simulink model "car_model_PIL"  (R2019b)
settings: Solver=ode23tb  StartTime=0.0  StopTime=30  RelTol=1e-3
InitFcn:
  | CommonVariables
  | Klqr5Velocities
undefined symbols (not defined in the file): A_1, A_2, A_3, A_4, A_5, B1_1, B1_2, B1_3, B1_4, B1_5, BattChrgMax, BattDischrgMax, BrkPrsMax, ChrgLmt_bpt, Disabled, DischrgLmt_bpt, Discovery, disk_abore, DLCXref, DLCYref, efficiency_table, F0z, h, Klqr1, Klqr2, Klqr3, Klqr4, Klqr5, MotSpd, MotTrq, mu_kinetic, Ndiff, num_pads, RegenBrkCutOff, RegenBrkSpd_bpt, Right, Rm, Serial, SOC_bpt, STM32F4, T_eff_bp, VEH, w_eff_bp
libraries: simulink x10, vehdynlibtire x8, vehdynlibsuspension x7, vehdynlibscenariocommon x5, autolibutils x4, sim3dlib x4, autolibmappedmotor x4, autolibshared x2, sharedtransform x2, vehdynlibviscommon x2, pil_lib x1, vehdynlibdriver x1
(part 2 of 7)

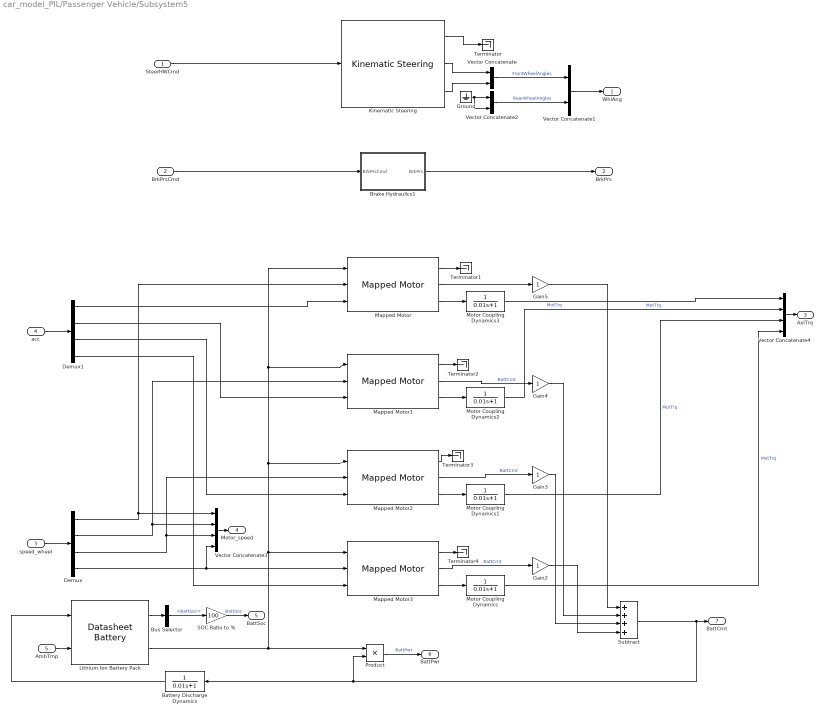
== system car_model_PIL/Passenger Vehicle/Subsystem5 ==
  SteerHWCmd : Inport
  BrkPrsCmd : Inport  Port=2  PortDimensions=4
  speed_wheel : Inport  Port=3
  "acc " : Inport  Port=4
  AmbTmp : Inport  Port=5
  Battery Discharge Dynamics : TransferFcn  Denominator=[0.01 1]
  Brake Hydraulics1 : Subsystem
  Bus Selector : BusSelector  OutputSignals=BattSoc
  Demux : Demux
  Demux1 : Demux
  Gain{2..5} (4 alike) : Gain
  Ground : Ground
  Kinematic Steering : vehdynlibsteering/Kinematic Steering  StrgType=Ackerman  StrgRatioType=Constant  Loc=Front  NrmlFctr=1  TrckWdth=1.922  WhlBase=(1.515+1.504)  Db=0  StrgRng=3*pi  StrgAngBpts="[-6.2832   -5.0265   -3.7699   -2.5133   -1.2566         0    1.2566    2.5133    3.7699    5.0265    6.2832]"  StrgRatioTbl=|  StrgRatio=18  StrgArmLngth=0.1  RckCsLngth=0.5  TieRodLngth=0.248128028933392  D=0.2  PnnRadius=0.0057  PnnRadiusTbl="[0.0055    0.0055    0.0056    0.0057    0.0057    0.0057    0.0057    0.0057    0.0056    0.0055    0.0055]"  RodLngth=0.1  ParaArmLngth=0.9  aMode=2
      | [13.5000   13.3750   13.2500   13.1250   13.0000   13.0000   13.0000   13.1250   13.2500   13.3750   13.5000
      | ]
      settings: SourceProductName=Vehicle Dynamics Blockset
  Lithium Ion Battery Pack : autolibdatasheetbattery/Datasheet Battery  CapacityCtrl=Parameter  OutputVlt=Unfiltered  BattChargeMax=BattChargeMax  Em=Em  CapLUTBp=CapLUTBp  RInt=RInt  BattTempBp=BattTempBp  CapSOCBp=CapSOCBp  Ns=Ns  Np=Np  BattCapInit=BattCapInit  Tc=1/1000  Vinit=3.75*72  RefBlkName='autolibdatasheetbattery/Datasheet Battery'
      settings: SourceProductName=Powertrain Blockset  SourceProductBaseCode=PW
  Mapped Motor{,1..3} (4 alike) : autolibmappedmotor/Mapped Motor  port_config=Speed  param_by=Maximum torque and power  w_t=[ 0 375 750 800 ]  T_t=[0.09 0.08 0.07 0]  torque_max=torque_max  power_max=power_max  Tc=Tc  param_loss=Tabulated efficiency data  eff=100  w_eff=375  T_eff=0.08  Piron=0  Pbase=0  w_eff_bp=w_eff_bp.*pi/30  T_eff_bp=T_eff_bp  Temp_eff_bp=[233.15 293.15 373.15]  losses_table=[1 2;3 4]  losses_table_3d=cat(3,[1.49 1.67 2.21 3.10; 0.42 0.69 1.14 2.03; 0.06 0.24 0.78 1.68; 0.42 0.69 1.14 2.03; 1.49 1.67 2.21 3.10],[1.49 1.67 2.21 3.10; 0.42 0.69 1.14 2.03; 0.06 0.24 0.78 1.68; 0.42 0.69 1.14 2.03; 1.49 1.67 2.21 3.10],[1.49 1.67 2.21 3.10; 0.42 0.69 1.14 2.03; 0.06 0.24 0.78 1.68; 0.42 0.69 1.14 2.03; 1.49 1.67 2.21 3.10])  efficiency_table=efficiency_table  efficiency_table_3d=cat(3,[95 95 95 95; 95 95 95 95; 95 95 95 95; 95 95 95 95; 95 95 95 95],[95 95 95 95; 95 95 95 95; 95 95 95 95; 95 95 95 95; 95 95 95 95],[95 95 95 95; 95 95 95 95; 95 95 95 95; 95 95 95 95; 95 95 95 95])  J=5e-6  b=1e-5  omega_o=0  T_t_extended=[0 0.07 0.08 0.09 0.08 0.07 0]  w_t_extended=[-800 -750 -375 0 375 750 800]  KLossIron=0  KLossCopper=0  x_w_eff_vec=[-1047.1975511966 -942.477796076938 -837.758040957278 -733.038285837618 -628.318530717959 -523.598775598299 -418.879020478639 -314.159265358979 -285.714285713875 -209.43951023932 -104.71975511966 0 104.71975511966 209.43951023932 285.714285713875 314.159265358979 418.879020478639 523.598775598299 628.318530717959 733.038285837618 837.758040957278 942.477796076938 1047.1975511966]  x_T_eff_vec=[-280 -260 -240 -220 -200 -180 -160 -140 -120 -100 -80 -60 -40 -20 0 20 40 60 80 100 120 140 160 180 200 220 240 260 280]  x_tmp_eff_vec=[-0.09 -0.06 -0.03 0 0.03 0.06 0.09]  x_losses_mat=[22069.9698961863 20493.5434750302 18917.117053874 17340.6906327178 15764.2642115617 14187.8377904055 12611.4113692493 11034.9849480932 9458.558526937 7882.13210578084 6305.70568462467 5463.63939754746 4654.21133865155 3695.99135716446 0 3141.59265358979 4188.79020478639 5026.54824574367 5864.30628670094 7330.38285837618 8796.45943005141 10262.5360017267 11728.6125734019 13194.6891450771 14660.7657167524 16126.8422884276 17592.9188601028 19058.9954317781 20525.0720034533;16844.2840149921 15641.1208710641 14437.9577271361 13234.7945832081 12031.6314392801 10828.4682953521 9625.30515142405 8422.14200749604 7218.97886356803 6015.81571964003 4812.65257571202 3609.48943178402 2837.5675580811 3326.39222144802 0 2827.43338823081 2638.93782901542 3392.92006587697 4523.8934211693 5654.86677646162 6785.84013175395 7916.81348704627 9047.7868423386 10178.7601976309 11309.7335529232 12440.7069082156 13571.6802635079 14702.6536188002 15833.6269740925;12345.907972002 11464.0574025733 10582.2068331446 9700.35626371584 8818.50569428713 7936.65512485842 7054.8045554297 6172.95398600099 5291.10341657228 4409.25284714356 3527.40227771485 3208.43505047468 2522.28227384987 2956.79308573157 0 2513.27412287184 2345.72251468038 3015.9289474462 3351.03216382911 4188.79020478639 5026.54824574366 5864.30628670094 6702.06432765822 7539.82236861549 8377.58040957277 9215.33845053005 10053.0964914873 10890.8545324446 11728.6125734019;10802.6694755017 10031.0502272516 9259.43097900148 8487.81173075136 7716.19248250124 6944.57323425111 6172.95398600099 5401.33473775087 4629.71548950074 3858.09624125062 3086.47699300049 2807.38066916535 2206.99698961863 2587.19395001512 0 2199.11485751286 2052.50720034533 2638.93782901542 2932.15314335047 3665.19142918809 4398.2297150257 5131.26800086332 5864.30628670094 6597.34457253856 7330.38285837617 8063.42114421379 8796.45943005141 9529.49771588903 10262.5360017266;9259.43097900149 8598.04305192995 7936.65512485842 7275.26719778688 6613.87927071535 5952.49134364381 5291.10341657228 4629.71548950074 3968.32756242921 3306.93963535767 3208.43505047468 2406.32628785601 1891.7117053874 2217.59481429868 0 1884.95559215388 1759.29188601028 2261.94671058465 3015.9289474462 3141.59265358979 3769.91118430775 4398.22971502571 5026.54824574366 5654.86677646162 6283.18530717958 6911.50383789754 7539.82236861549 8168.14089933345 8796.45943005141;7716.19248250124 7165.03587660829 6613.87927071535 6062.7226648224 5511.56605892946 4960.40945303651 4409.25284714356 3858.09624125062 3306.93963535767 2755.78302946473 2673.69587539557 2005.27190654668 1576.42642115617 1847.99567858223 0 1570.7963267949 1466.07657167524 1884.95559215387 2513.27412287183 2617.99387799149 3141.59265358979 3665.19142918809 4188.79020478639 4712.38898038468 5235.98775598298 5759.58653158128 6283.18530717958 6806.78408277788 7330.38285837618;7486.34845110759 6951.60927602848 6416.87010094936 5882.13092587025 5347.39175079114 4812.65257571202 4277.91340063291 3743.17422555379 3208.43505047468 2673.69587539557 2138.95670031645 1604.21752523734 1261.14113692493 1478.39654286579 0 1256.63706143592 1172.86125734019 1507.9644737231 2010.61929829747 2513.27412287183 3015.9289474462 3518.58377202056 4021.23859659493 4523.8934211693 5026.54824574366 5529.20307031803 6031.8578948924 6534.51271946676 7037.16754404113;9773.84381116825 9075.71211037052 8377.58040957279 7679.44870877505 5463.63939754746 4917.27545779272 4370.91151803797 3310.49548442795 2837.5675580811 2364.63963173425 1891.7117053874 1639.09181926424 1092.72787950949 1108.79740714934 0 942.477796076938 1005.30964914873 1507.9644737231 1759.29188601028 2199.11485751285 2638.93782901542 3078.760800518 4021.23859659493 4523.8934211693 5026.54824574367 6911.50383789754 7539.8223686155 8168.14089933346 8796.45943005142;8888.88888887612 8253.9682539564 7619.04761903668 6984.12698411695 4968.94409937174 4472.04968943457 3975.15527949739 3478.26086956022 2981.36645962304 2484.47204968587 1987.5776397487 ...(+6498 chars)]  x_losses_mat_3d=[37.8947368421052 25.2631578947368 12.6315789473684 0 12 24 36;18.9473684210526 12.6315789473684 6.3157894736842 0 5.99999999999999 12 18;0 0 0 0 0 0 0;18 12 5.99999999999999 0 6.3157894736842 12.6315789473684 18.9473684210526;36 24 12 0 12.6315789473684 25.2631578947368 37.8947368421052]  CalLossMapData={}  CalLossWithTempMapData={}  aMode=aMode  RefBlkName='autolibmappedmotor/Mapped Motor'
      settings: SourceProductName=Powertrain Blockset  SourceProductBaseCode=PW
  Motor Coupling Dynamics{,1..3} (4 alike) : TransferFcn  Denominator=[0.01 1]
  Product : Product
  SOC Ratio to % : Gain  Gain=100
  Subtract : Sum  Inputs=++++
  Terminator{,1..4} (5 alike) : Terminator
  Vector Concatenate : Concatenate
  Vector Concatenate1 : Concatenate
  Vector Concatenate2 : Concatenate
  Vector Concatenate3 : Concatenate  NumInputs=4
  Vector Concatenate4 : Concatenate  NumInputs=4
  WhlAng : Outport  Unit=rad  VectorParamsAs1DForOutWhenUnconnected=off
  BrkPrs : Outport  Port=2  PortDimensions=4  VectorParamsAs1DForOutWhenUnconnected=off
  AxlTrq : Outport  Port=3  VectorParamsAs1DForOutWhenUnconnected=off
  Motor_speed : Outport  Port=4  VectorParamsAs1DForOutWhenUnconnected=off
  BattSoc : Outport  Port=5  VectorParamsAs1DForOutWhenUnconnected=off
  BattPwr : Outport  Port=6  VectorParamsAs1DForOutWhenUnconnected=off
  BattCrnt : Outport  Port=7  VectorParamsAs1DForOutWhenUnconnected=off
  wires:
  SteerHWCmd/1 -> Kinematic Steering/1
  Kinematic Steering/1 -> Terminator/1
  Vector Concatenate2/1 -> Vector Concatenate1/2  "RearWheelAngles"
  Vector Concatenate1/1 -> WhlAng/1
  BrkPrsCmd/1 -> Brake Hydraulics1/1(BrkPrsCmd)
  Brake Hydraulics1/1(BrkPrs) -> BrkPrs/1
  Kinematic Steering/2 -> Vector Concatenate/1
  Kinematic Steering/3 -> Vector Concatenate/2
  Vector Concatenate/1 -> Vector Concatenate1/1  "FrontWheelAngles"
  Mapped Motor3/3 -> Motor Coupling Dynamics/1
  Battery Discharge Dynamics/1 -> Lithium Ion Battery Pack/1
  Product/1 -> BattPwr/1  "BattPwr"
  Motor Coupling Dynamics/1 -> Vector Concatenate4/4  "MotTrq"
  AmbTmp/1 -> Lithium Ion Battery Pack/2
  SOC Ratio to %/1 -> BattSoc/1  "BattSoc"
  Lithium Ion Battery Pack/2 -> Product/1, Mapped Motor3/1, Mapped Motor2/1, Mapped Motor1/1, Mapped Motor/1
  Demux1/4 -> Mapped Motor3/3
  Demux1/3 -> Mapped Motor2/3
  Mapped Motor2/3 -> Motor Coupling Dynamics1/1
  Motor Coupling Dynamics1/1 -> Vector Concatenate4/3  "MotTrq"
  Demux1/2 -> Mapped Motor1/3
  Motor Coupling Dynamics2/1 -> Vector Concatenate4/2  "MotTrq"
  Demux1/1 -> Mapped Motor/3
  Motor Coupling Dynamics3/1 -> Vector Concatenate4/1  "MotTrq"
  Vector Concatenate4/1 -> AxlTrq/1
  Subtract/1 -> Product/2, Battery Discharge Dynamics/1, BattCrnt/1
  Mapped Motor2/2 -> Gain3/1  "BattCrnt"
  Mapped Motor1/2 -> Gain4/1  "BattCrnt"
  Mapped Motor3/2 -> Gain2/1  "BattCrnt"
  Gain2/1 -> Subtract/4
  Gain3/1 -> Subtract/3
  Gain4/1 -> Subtract/2
  Gain5/1 -> Subtract/1
  "acc "/1 -> Demux1/1
  Mapped Motor/1 -> Terminator1/1
  Mapped Motor/3 -> Motor Coupling Dynamics3/1
  Mapped Motor/2 -> Gain5/1
  Mapped Motor1/3 -> Motor Coupling Dynamics2/1
  Mapped Motor1/1 -> Terminator2/1
  Mapped Motor2/1 -> Terminator3/1
  Mapped Motor3/1 -> Terminator4/1
  Vector Concatenate3/1 -> Motor_speed/1
  speed_wheel/1 -> Demux/1
  Demux/1 -> Mapped Motor/2, Vector Concatenate3/1
  Demux/2 -> Vector Concatenate3/2, Mapped Motor1/2
  Demux/3 -> Mapped Motor2/2, Vector Concatenate3/3
  Demux/4 -> Vector Concatenate3/4, Mapped Motor3/2
  Lithium Ion Battery Pack/1 -> Bus Selector/1
  Bus Selector/1 -> SOC Ratio to %/1  "<BattSoc>"
  Ground/1 -> Vector Concatenate2/2, Vector Concatenate2/1

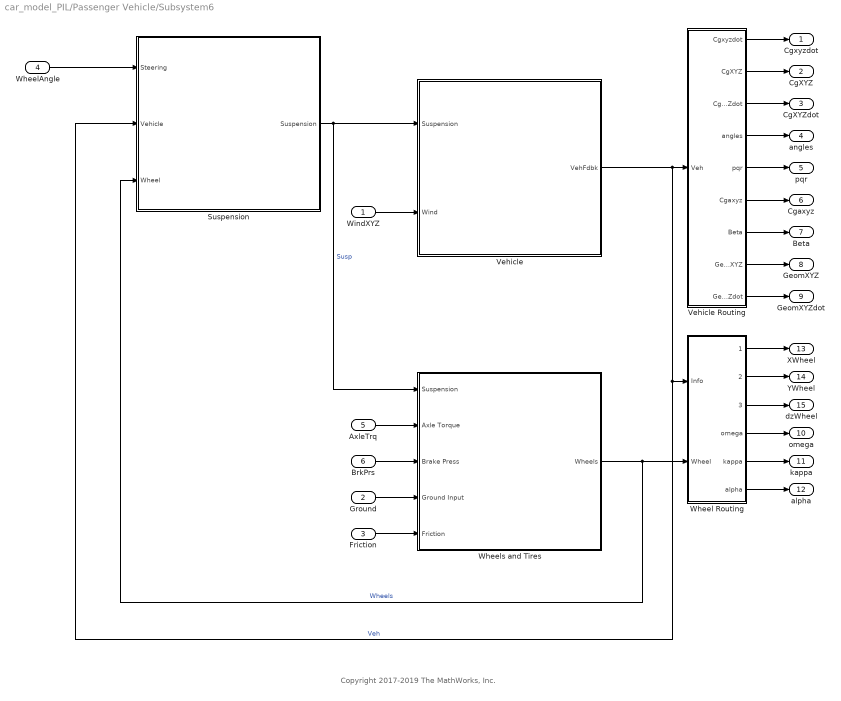
== system car_model_PIL/Passenger Vehicle/Subsystem6 ==
  note: Copyright 2017-2019 The MathWorks, Inc.
  WindXYZ : Inport  Unit=m/s  PortDimensions=3
  Ground : Inport  Port=2  Unit=m  PortDimensions=4
  Friction : Inport  Port=3  Unit=1  PortDimensions=4
  WheelAngle : Inport  Port=4  Unit=rad  PortDimensions=4
  AxleTrq : Inport  Port=5  Unit=N*m  PortDimensions=4
  BrkPrs : Inport  Port=6  PortDimensions=4
  Suspension : Subsystem  VariantControlMode=Label  Variant=on  LabelModeActiveChoice=3
      mask Display:
      | switch str2num(get_param(gcb,'ActiveVariant'))
      |     case 1
      |         image('suspdw.png');
      |     case 2
      |         image([imread('suspindmap.png');imread('suspsamap.png')]);
      |     case 3
      |          image([imread('suspmacp.png');imread('suspsacoil.png')]);
      |     case 4
      |          image('suspmacp.png');
      |     case 5
      |          image('suspindmap.png');
      | end
  Vehicle : Subsystem
      mask Display: image('6dofcar.png');
  Vehicle Routing : Subsystem
  Wheel Routing : Subsystem
  Wheels and Tires : Subsystem
      mask Display: image('wheel3dof.png')
  Cgxyzdot : Outport  VectorParamsAs1DForOutWhenUnconnected=off
  CgXYZ : Outport  Port=2  VectorParamsAs1DForOutWhenUnconnected=off
  CgXYZdot : Outport  Port=3  VectorParamsAs1DForOutWhenUnconnected=off
  angles : Outport  Port=4  VectorParamsAs1DForOutWhenUnconnected=off
  pqr : Outport  Port=5  VectorParamsAs1DForOutWhenUnconnected=off
  Cgaxyz : Outport  Port=6  VectorParamsAs1DForOutWhenUnconnected=off
  Beta : Outport  Port=7  VectorParamsAs1DForOutWhenUnconnected=off
  GeomXYZ : Outport  Port=8  VectorParamsAs1DForOutWhenUnconnected=off
  GeomXYZdot : Outport  Port=9  VectorParamsAs1DForOutWhenUnconnected=off
  omega : Outport  Port=10  PortDimensions=4  VectorParamsAs1DForOutWhenUnconnected=off
  kappa : Outport  Port=11  PortDimensions=4  VectorParamsAs1DForOutWhenUnconnected=off
  alpha : Outport  Port=12  PortDimensions=4  VectorParamsAs1DForOutWhenUnconnected=off
  XWheel : Outport  Port=13  VectorParamsAs1DForOutWhenUnconnected=off
  YWheel : Outport  Port=14  VectorParamsAs1DForOutWhenUnconnected=off
  dzWheel : Outport  Port=15  PortDimensions=4  VectorParamsAs1DForOutWhenUnconnected=off
  wires:
  Vehicle Routing/7(Beta) -> Beta/1
  Vehicle/1(VehFdbk) -> Suspension/2(Vehicle), Wheel Routing/1(Info), Vehicle Routing/1(Veh)  "Veh"
  Friction/1 -> Wheels and Tires/5(Friction)
  WheelAngle/1 -> Suspension/1(Steering)
  WindXYZ/1 -> Vehicle/2(Wind)
  Wheels and Tires/1(Wheels) -> Suspension/3(Wheel), Wheel Routing/2(Wheel)  "Wheels"
  Vehicle Routing/2(CgXYZ) -> CgXYZ/1
  AxleTrq/1 -> Wheels and Tires/2(Axle Torque)
  Vehicle Routing/4(angles) -> angles/1
  Wheel Routing/1(XWheel) -> XWheel/1
  Vehicle Routing/1(Cgxyzdot) -> Cgxyzdot/1
  Wheel Routing/2(YWheel) -> YWheel/1
  Suspension/1(Suspension) -> Wheels and Tires/1(Suspension), Vehicle/1(Suspension)  "Susp"
  Wheel Routing/4(omega) -> omega/1
  Vehicle Routing/6(Cgaxyz) -> Cgaxyz/1
  Vehicle Routing/5(pqr) -> pqr/1
  BrkPrs/1 -> Wheels and Tires/3(Brake Press)
  Vehicle Routing/8(GeomXYZ) -> GeomXYZ/1
  Vehicle Routing/9(GeomXYZdot) -> GeomXYZdot/1
  Ground/1 -> Wheels and Tires/4(Ground Input)
  Wheel Routing/3(ZWheel) -> dzWheel/1
  Wheel Routing/5(kappa) -> kappa/1
  Vehicle Routing/3(CgXYZdot) -> CgXYZdot/1
  Wheel Routing/6(alpha) -> alpha/1

== system car_model_PIL/Reference Generator/3D Engine ==
  note: 1) Add Subsystem or Model blocks as valid variant choices.
      | 2) You cannot connect blocks at this level. At simulation, connectivity is automatically
      | determined, based on the active variant and port name matching.
  VehFdbk : Inport
  3D Engine : Subsystem  VariantControl=1
  3D Engine Disabled : Subsystem  VariantControl=0

== system car_model_PIL/Reference Generator/Reference Generator ==
  "VehFdbk " : Inport
  Constant Radius : Subsystem  AncestorBlock=vehdynlibscenariocommon/Constant Radius  VariantControl=4  mask{t_start=t_start, xdot_r=xdot_r, xdotUnit=mph, R=R, turnDirMask=Right, ay_max=cr_ay_max, ay_stop=off, Parameter6=2}
      mask prompts: t_start "Maneuver start time, t_start [s]:"; xdot_r "Longitudinal velocity reference, xdot_r:"; xdotUnit "Longitudinal velocity reference units, xdotUnit []:"; R "Radius value, R [m]:"; turnDirMask "Turn direction"; ay_max "Lateral acceleration absolute threshold, ay_max [g]:"; ay_stop "Stop simulation at lateral acceleration threshold"
      mask TypeOptions xdotUnit: Longitudinal Velocity Reference/Input Units/Unit
      mask TypeOptions R: Constant Radius/Value
      mask TypeOptions turnDirMask: Constant Radius/turnDirMask
  Double Lane Change : Subsystem  VariantControl=0
  Increasing Steer : Subsystem  VariantControl=1
  Sine with Dwell : Subsystem  VariantControl=3
  Swept Sine : Subsystem  VariantControl=2
  " Vis" : Outport  VectorParamsAs1DForOutWhenUnconnected=off
  " Ref" : Outport  Port=2  VectorParamsAs1DForOutWhenUnconnected=off
  " Fdbk" : Outport  Port=3  VectorParamsAs1DForOutWhenUnconnected=off

== system car_model_PIL/Visualization/ISO 15037-1:2006 ==
  VehFdbk : Inport
  Cntrl : Inport  Port=2
  Disabled : Subsystem  VariantControl=0
  Enabled : Subsystem  VariantControl=1

== system car_model_PIL/Visualization/Scope Type ==
  "VehFdbk " : Inport
  Cntrl : Inport  Port=2
  "Vis " : Inport  Port=3
  DLC : Subsystem  VariantControl=1
  None : Subsystem  VariantControl=0
  XYZ : Subsystem  VariantControl=2
  " Ref" : Outport  VectorParamsAs1DForOutWhenUnconnected=off

== system car_model_PIL/Visualization/Vehicle XY Plotter ==
  "VehFdbk " : Inport
  "Ref " : Inport  Port=2
  XY View : Subsystem  VariantControl=0
  XY View Ref : Subsystem  VariantControl=1

== system car_model_PIL/Controllers/Accel Pedal to Traction Wheel Torque Request/Apply ESP control ==
  Beta : Inport
  Omega : Inport  Port=2
  Vspd : Inport  Port=3
  K1 : Gain  Gain=Klqr1  Multiplication=Matrix(K*u)
  K2 : Gain  Gain=Klqr2  Multiplication=Matrix(K*u)
  K3 : Gain  Gain=Klqr3  Multiplication=Matrix(K*u)
  K4 : Gain  Gain=Klqr4  Multiplication=Matrix(K*u)
  K5 : Gain  Gain=Klqr5  Multiplication=Matrix(K*u)
  Switch control action : MATLAB Function  TreatAsAtomicUnit=on
  Vector Concatenate : Concatenate
  dWhlSpd : Outport
  wires:
  Beta/1 -> Vector Concatenate/1
  Vector Concatenate/1 -> Switch control action/7(x), K5/1, K4/1, K3/1, K2/1, K1/1
  K5/1 -> Switch control action/6(contr5)
  Omega/1 -> Vector Concatenate/2
  K1/1 -> Switch control action/2(contr1)
  K3/1 -> Switch control action/4(contr3)
  K4/1 -> Switch control action/5(contr4)
  K2/1 -> Switch control action/3(contr2)
  Vspd/1 -> Switch control action/1(V)
  Switch control action/1(u) -> dWhlSpd/1

== system car_model_PIL/Controllers/Accel Pedal to Traction Wheel Torque Request/Signals to states ==
  Beta : Inport
  YawRate : Inport  Port=2
  WhlAng : Inport  Port=3
  Vspd : Inport  Port=4
  Constant : Constant  Value=[A_1;A_2;A_3;A_4;A_5]  VectorParams1D=off
  Constant1 : Constant  Value=[B1_1;B1_2;B1_3;B1_4;B1_5]  VectorParams1D=off
  Demux : Demux  Outputs=2
  Gain : Gain  Gain=1/2
  Subtract : Sum  Inputs=+-
  Subtract1 : Sum  Inputs=-+
  Sum of Elements : Sum  Inputs=+
  equilibrium point : MATLAB Function  TreatAsAtomicUnit=on
  Beta_state : Outport
  Omega_state : Outport  Port=2
  wires:
  Subtract/1 -> Beta_state/1
  Beta/1 -> Subtract/1
  Subtract1/1 -> Omega_state/1
  YawRate/1 -> Subtract1/2
  WhlAng/1 -> Sum of Elements/1
  Sum of Elements/1 -> Gain/1
  equilibrium point/1(x_eq) -> Demux/1
  Demux/1 -> Subtract/2
  Demux/2 -> Subtract1/1
  Gain/1 -> equilibrium point/1(delta)
  Vspd/1 -> equilibrium point/2(V)
  Constant/1 -> equilibrium point/3(A_mat)
  Constant1/1 -> equilibrium point/4(B_mat)

== system car_model_PIL/Controllers/Accel Pedal to Traction Wheel Torque Request/Virtual Ackerman differential ==
  note: Wheels are organized as:
      |
      | 1 ------------ 2
      | |
      | |
      | |
      | |
      | 3 ------------ 4
      |
      | But output inverting 3 and 4
      | (for easier integration)
  WhlAng : Inport
  RefSpd : Inport  Port=2
  Abs : Abs
  Cos : Trigonometry  Operator=cos
  Demux : Demux
  Divide : Product  Inputs=*/
  Divide1 : Product  Inputs=*/
  Divide2 : Product  Inputs=*/
  Fcn : Fcn  Expr=sqrt( ((u(4) + u(5))/ 2)^2 + u(1)^2 )
  Mux : Mux
  Product : Product
  Product1 : Product
  Saturation RefSpd : Saturate  UpperLimit=120  LowerLimit=-120
  Saturation WhlAnd : Saturate  UpperLimit=pi*5/12  LowerLimit=-pi*5/12
  Saturation WhlSpd : Saturate  UpperLimit=600  LowerLimit=-600
  Sin : Trigonometry
  Sum : Sum  Inputs=+-|
  Vector Concatenate1 : Concatenate
  Vector Concatenate2 : Concatenate
  pi half : Constant  Value=pi/2
  wheel base : Constant  Value=VEH.FrontAxlePositionfromCG+VEH.RearAxlePositionfromCG
  wheel base1 : Constant  Value=VEH.RearAxlePositionfromCG
  wheel radius : Constant  Value=VEH.WheelRadius
  WhlSpd : Outport
  wires:
  Sin/1 -> Product1/2
  Cos/1 -> Divide/2
  wheel base/1 -> Divide/1
  Divide/1 -> Vector Concatenate2/1, Product1/1  "[d1; d2]"
  Vector Concatenate1/1 -> Fcn/1
  Fcn/1 -> Divide1/2  "d_v"
  Divide1/1 -> Product/1  "w_v"
  Divide2/1 -> Product/2  "d_x/r_w"
  wheel radius/1 -> Divide2/2
  pi half/1 -> Sum/1
  Sum/1 -> Sin/1, Cos/1
  Product1/1 -> Vector Concatenate2/2  "[d3; d4]"
  Vector Concatenate2/1 -> Divide2/1, Vector Concatenate1/2  "[d1; d2; d3; d4]"
  Abs/1 -> Sum/2
  Saturation WhlAnd/1 -> Abs/1
  WhlAng/1 -> Saturation WhlAnd/1  "[delta1; delta2]"
  Saturation RefSpd/1 -> Divide1/1
  RefSpd/1 -> Saturation RefSpd/1
  Product/1 -> Saturation WhlSpd/1  "[w1; w2; w3; w4]"
  Saturation WhlSpd/1 -> Demux/1
  Mux/1 -> WhlSpd/1
  Demux/1 -> Mux/1
  Demux/2 -> Mux/2
  Demux/4 -> Mux/3
  Demux/3 -> Mux/4
  wheel base1/1 -> Vector Concatenate1/1

== system car_model_PIL/Controllers/Accel Pedal to Traction Wheel Torque Request1/__InputSSForSFun__ ==
  AccelPdl : Inport
  WhlAng : Inport  Port=2
  xdot : Inport  Port=3
  ydot : Inport  Port=4
  YawRate : Inport  Port=5
  MotSpd : Inport  Port=6
  __UniqueOutportName__1__ : Outport
  __UniqueOutportName__2__ : Outport  Port=2
  __UniqueOutportName__3__ : Outport  Port=3
  __UniqueOutportName__4__ : Outport  Port=4
  __UniqueOutportName__5__ : Outport  Port=5
  __UniqueOutportName__6__ : Outport  Port=6
  wires:
  AccelPdl/1 -> __UniqueOutportName__1__/1
  WhlAng/1 -> __UniqueOutportName__2__/1
  xdot/1 -> __UniqueOutportName__3__/1
  ydot/1 -> __UniqueOutportName__4__/1
  YawRate/1 -> __UniqueOutportName__5__/1
  MotSpd/1 -> __UniqueOutportName__6__/1

== system car_model_PIL/Controllers/Accel Pedal to Traction Wheel Torque Request1/__OutputSSForSFun__ ==
  __UniqueInportName__1__ : Inport
  TrqCmd : Outport  VectorParamsAs1DForOutWhenUnconnected=off
  wires:
  __UniqueInportName__1__/1 -> TrqCmd/1

== system car_model_PIL/Controllers/Motor Torque Arbitration and Power Management/Power Management ==
  note: Power Management algorithm:
      | - Estimate Elec power based on mech power using efficiency map
      | - Check if Elec power is within battery power limits
      | - If power within limit , use motor torque command
      | - If power limit exceeded, use limited motor torque
      | - For low Mot Spd, MotPwrReq will be a small number.  Pass through torque command until Mot Spd > 2.
  BattPwrDischrgLmt : Inport
  BattPwrChrgLmt : Inport  Port=2
  MotSpd : Inport  Port=3
  MotTrqCmd : Inport  Port=4
  Abs : Abs
  Check Within Limits : Subsystem
  Compare To Constant : simulink/Logic and Bit Operations/Compare To Constant  relop=<  const=2  OutDataTypeStr=boolean
  ElecToMechPwr : Product  Inputs=*/
  Mech to Elec Power Estimate : Subsystem
  MechPwrToTrq : Product  Inputs=*/
  Switch : Switch  Criteria=u2 > Threshold
  Switch1 : Switch  Criteria=u2 > Threshold
  Torque Limit : Subsystem
  div0protect - poly : autolibutils/div0protect - poly  thresh=2  aMode=aMode
      settings: SourceProductName=Powertrain Blockset  SourceProductBaseCode=PW
  MotTrqCmdFinal : Outport  VectorParamsAs1DForOutWhenUnconnected=off
  wires:
  MotSpd/1 -> Abs/1, Torque Limit/2(MotSpd), div0protect - poly/1, Mech to Elec Power Estimate/2(MotSpd)
  MotTrqCmd/1 -> Switch/1, Switch1/1, Mech to Elec Power Estimate/1(MotTrqCmd)
  div0protect - poly/1 -> MechPwrToTrq/2
  Mech to Elec Power Estimate/2(Eff2k) -> ElecToMechPwr/2
  ElecToMechPwr/1 -> MechPwrToTrq/1
  MechPwrToTrq/1 -> Switch/3
  Torque Limit/1(MotTrqCmd) -> MotTrqCmdFinal/1
  BattPwrDischrgLmt/1 -> Check Within Limits/1(up)
  Mech to Elec Power Estimate/1(MotPwrElecReq) -> Check Within Limits/2(u)
  BattPwrChrgLmt/1 -> Check Within Limits/3(lo)
  Check Within Limits/2(y) -> ElecToMechPwr/1
  Switch/1 -> Switch1/3
  Check Within Limits/1(InLimit) -> Switch/2
  Switch1/1 -> Torque Limit/1(MotTrq)
  Abs/1 -> Compare To Constant/1
  Compare To Constant/1 -> Switch1/2

== system car_model_PIL/Controllers/Regen Braking Control/Parallel Regen Braking ==
  VehSpd : Inport
  MotSpd : Inport  Port=2
  "BrkPrsReq " : Inport  Port=3
  BattSoc : Inport  Port=4
  ChrgLmt : Lookup_n-D  NumberOfTableDimensions=1  BreakpointsForDimension1=[0:10:100]  Table=[1 1 1 1 1 1 1 1 0.7 0.35 0]  ExtrapMethod=Clip  UseLastTableValue=on  InternalRulePriority=Speed  RndMeth=Simplest  InputSameDT=on
  Gain : Gain  Gain=-1
  MaxMotorTrqVsSpd : Lookup_n-D  NumberOfTableDimensions=1  BreakpointsForDimension1=MotSpd  Table=MotTrq  ExtrapMethod=Clip  UseLastTableValue=on  InternalRulePriority=Speed  OutDataTypeStr=Inherit: Inherit from 'Table data'  RndMeth=Simplest  InputSameDT=on
  Product1 : Product
  Product3 : Product
  RegenBrakingCutoff : Lookup_n-D  NumberOfTableDimensions=1  BreakpointsForDimension1=[2.2 4.5]  Table=[0 1]  ExtrapMethod=Clip  UseLastTableValue=on  InternalRulePriority=Speed  RndMeth=Simplest  InputSameDT=on
  rads_to_rpm : Gain  Gain=30/pi
  " MotTrqCmdRegen" : Outport  VectorParamsAs1DForOutWhenUnconnected=off
  " BrkCmd" : Outport  Port=2  VectorParamsAs1DForOutWhenUnconnected=off
  wires:
  Gain/1 -> " MotTrqCmdRegen"/1
  BattSoc/1 -> ChrgLmt/1
  Product3/1 -> Gain/1  "MotTrqRegen"
  Product1/1 -> Product3/2  "RegenFactor"
  RegenBrakingCutoff/1 -> Product1/1
  VehSpd/1 -> RegenBrakingCutoff/1
  ChrgLmt/1 -> Product1/2
  MaxMotorTrqVsSpd/1 -> Product3/1  "MotTrqMax"
  rads_to_rpm/1 -> MaxMotorTrqVsSpd/1
  MotSpd/1 -> rads_to_rpm/1
  "BrkPrsReq "/1 -> " BrkCmd"/1  "BrkPrsReq"

== system car_model_PIL/Controllers/Regen Braking Control/Series Regen Braking ==
  note: - Total brake torque request based on brake pressure and parameters of disc brakes
      | - Use as much regenerative motor braking as possible
      | - Any braking torque request that cannot be provided by the motor, will be provided by the friction brakes
  note: T / 4 brakes*(muk*pi*Ba^2*Rm*Npads/4)
  note: 4 brakes*(muk*pi*Ba^2*Rm*Npads/4)*P
  VehSpd : Inport
  MotSpd : Inport  Port=2
  "BrkPrsReq " : Inport  Port=3
  BattSoc : Inport  Port=4
  ChrgLmt : Lookup_n-D  NumberOfTableDimensions=1  BreakpointsForDimension1=SOC_bpt  Table=ChrgLmt_bpt  ExtrapMethod=Clip  UseLastTableValue=on  InternalRulePriority=Speed  RndMeth=Simplest  InputSameDT=on
  Constant : Constant  Value=4*(mu_kinetic*pi*disk_abore^2*Rm*num_pads/4)
  Constant1 : Constant  Value=4*(mu_kinetic*pi*disk_abore^2*Rm*num_pads/4)
  Gain : Gain  Gain=-1
  MaxMotTrqVsSpd : Lookup_n-D  NumberOfTableDimensions=1  BreakpointsForDimension1=MotSpd  Table=MotTrq  ExtrapMethod=Clip  UseLastTableValue=on  InternalRulePriority=Speed  OutDataTypeStr=Inherit: Inherit from 'Table data'  RndMeth=Simplest  InputSameDT=on
  MinMax : MinMax  Inputs=2
  MotTrqReflectedToWheels : Gain  Gain=Ndiff
  Negative 5 : Saturate  UpperLimit=inf  LowerLimit=0
  Product1 : Product
  Product2 : Product
  Product3 : Product
  Product4 : Product  Inputs=*/
  RegenBrakingCutoff : Lookup_n-D  NumberOfTableDimensions=1  BreakpointsForDimension1=RegenBrkSpd_bpt  Table=RegenBrkCutOff  ExtrapMethod=Clip  UseLastTableValue=on  InternalRulePriority=Speed  RndMeth=Simplest  InputSameDT=on
  Subtract : Sum  Inputs=+-
  WhlTrqReflectedToMot : Gain  Gain=1/Ndiff
  rads_to_rpm : Gain  Gain=30/pi
  " MotTrqCmdRegen" : Outport  VectorParamsAs1DForOutWhenUnconnected=off
  " BrkCmd" : Outport  Port=2  VectorParamsAs1DForOutWhenUnconnected=off
  wires:
  Product3/1 -> WhlTrqReflectedToMot/1, Subtract/2  "MotTrqRegenWhl"
  Product4/1 -> " BrkCmd"/1
  Constant1/1 -> Product4/2
  Constant/1 -> Product2/2
  "BrkPrsReq "/1 -> Product2/1  "BrkPrsReq"
  rads_to_rpm/1 -> MaxMotTrqVsSpd/1
  MaxMotTrqVsSpd/1 -> MotTrqReflectedToWheels/1  "MotTrqMax"
  Product2/1 -> MinMax/1, Subtract/1  "BrkTrqReqTotal"
  MinMax/1 -> Product3/1  "min"
  ChrgLmt/1 -> Product1/2
  VehSpd/1 -> RegenBrakingCutoff/1
  RegenBrakingCutoff/1 -> Product1/1
  Product1/1 -> Product3/2  "RegenFactor"
  Subtract/1 -> Negative 5/1
  BattSoc/1 -> ChrgLmt/1
  Negative 5/1 -> Product4/1  "BrkTrqFric"
  MotSpd/1 -> rads_to_rpm/1
  MotTrqReflectedToWheels/1 -> MinMax/2  "MotTrqMaxWhls"
  WhlTrqReflectedToMot/1 -> Gain/1
  Gain/1 -> " MotTrqCmdRegen"/1  "MotTrqCmdRegen"

== system car_model_PIL/Driver Commands/Driver Commands/Longitudinal Driver ==
  VehRef : Inport
  VehFdbk : Inport  Port=2
  Bus Creator1 : BusCreator  Inputs=4
  Bus Selector : BusSelector  OutputSignals=Body.xdot
  Bus Selector1 : BusSelector  OutputSignals=Steer,LngRef
  Dead Zone : DeadZone  LowerValue=-.1  UpperValue=.1  SaturateOnIntegerOverflow=on
  Ground : Ground
  Longitudinal Driver : autolibshared/Longitudinal Driver  cntrlType=Predictive  shftType=None  velUnits=m/s  gearOut=on  Kp=5  Ki=5  Kff=.1  Kg=0  VehVelVec=[0 100]  KffVec=[.1 .1]  KpVec=[10 10]  KiVec=[5 5]  KgVec=[0 0]  m=VEH.Mass  Kpt=3000  tau=.5  L=3  aR=200  bR=2.5  cR=.5  g=9.81  vnom=5  Kaw=1  tauerr=.1  tauPt=2  GearInit=0  tShift=.1  pdlVec=[0.1 0.4 0.5 0.9]  upShftTbl=[-1 12.9375 26.4375 39.9375 51.18749999999999 62.4375 72.84375 83.25;-1 16.3125 29.8125 43.3125 54.5624 65.8125 76.78125 87.75;-1 19.6875 33.1875 46.68749999999999 57.9375 69.1875 80.71875 92.25;-1 33 52.5 77.25 100.5 138.75 161.875 185]  dwnShftTbl=[1 9.5625 23.0625 36.5625 47.8125 59.0625 68.90625 78.75;1 12.9375 26.4375 39.9375 51.18749999999999 62.4375 72.84375 83.25;1 16.3125 29.8125 43.3125 54.562499 65.8125 76.78125 87.75;1 19.6875 33.1875 46.68749999999999 57.9375 69.1875 80.71875 92.25]  tClutch=.5  tRev=.5  tPark=120  aMode=2  UpGearVec="[0  1  2  3  4  5  6  7]"  DownGearVec="[1  2  3  4  5  6  7  8]"
      settings: SourceProductName=Powertrain Blockset  SourceProductBaseCode=PW
  Terminator3 : Terminator
  Unit Conversion : UnitConversion
  Driver : Outport  VectorParamsAs1DForOutWhenUnconnected=off
  wires:
  Dead Zone/1 -> Longitudinal Driver/2
  Bus Creator1/1 -> Driver/1
  Unit Conversion/1 -> Bus Creator1/1  "Steer"
  Longitudinal Driver/3 -> Bus Creator1/3  "Brake"
  Longitudinal Driver/1 -> Terminator3/1
  Bus Selector1/2 -> Longitudinal Driver/1  "<LngRef>"
  VehRef/1 -> Bus Selector1/1
  VehFdbk/1 -> Bus Selector/1
  Bus Selector/1 -> Dead Zone/1  "<xdot>"
  Longitudinal Driver/2 -> Bus Creator1/2  "Accel"
  Ground/1 -> Longitudinal Driver/3
  Longitudinal Driver/4 -> Bus Creator1/4  "Gear"
  Bus Selector1/1 -> Unit Conversion/1  "<Steer>"

== system car_model_PIL/Driver Commands/Driver Commands/Open Loop Constant Radius ==
  VehFdbk : Inport
  SteerCmd : Inport  Port=2
  Accel : Inport  Port=3
  Brake : Inport  Port=4
  Gear : Inport  Port=5
  Bus Creator1 : BusCreator  Inputs=4
  Terminator : Terminator
  Unit Conversion{,1..3} (4 alike) : UnitConversion
  Wheel Angle Limit * Steer Ratio : Gain  Gain=40*pi/180*18
  Driver : Outport  VectorParamsAs1DForOutWhenUnconnected=off
  wires:
  Unit Conversion3/1 -> Bus Creator1/4  "Gear"
  Unit Conversion2/1 -> Bus Creator1/3  "Brake"
  Wheel Angle Limit * Steer Ratio/1 -> Bus Creator1/1  "Steer"
  Bus Creator1/1 -> Driver/1
  Unit Conversion/1 -> Wheel Angle Limit * Steer Ratio/1  "SteerCmd"
  Accel/1 -> Unit Conversion1/1
  VehFdbk/1 -> Terminator/1
  SteerCmd/1 -> Unit Conversion/1
  Unit Conversion1/1 -> Bus Creator1/2  "Accel"
  Brake/1 -> Unit Conversion2/1
  Gear/1 -> Unit Conversion3/1

== system car_model_PIL/Driver Commands/Driver Commands/Predictive Driver ==
  VehRef : Inport
  VehFdbk : Inport  Port=2
  Bus Creator1 : BusCreator  Inputs=4
  Bus Selector : BusSelector  OutputSignals=Body.xdot,Body.Y,Body.ydot,Body.psi,Body.r
  Bus Selector1 : BusSelector  OutputSignals=LngRef,LtrlRef,ThrotKill
  Constant : Constant  Value=0
  Dead Zone : DeadZone  LowerValue=-.5  UpperValue=.5  ZeroCross=off  SaturateOnIntegerOverflow=on
  Dead Zone1 : DeadZone  LowerValue=-1e-2  UpperValue=1e-2  ZeroCross=off  SaturateOnIntegerOverflow=on
  Ground : Ground
  Linear Predictive Driver : vehdynlibdriver/Predictive Driver  cntrlType=Predictive  shftType=Reverse, Neutral, Drive  velUnits=m/s  gearOut=on  Kp=3  Ki=1  Kff=1  Kg=0  VehVelVec=[0 100]  KffVec=[.1 .1]  KpVec=[10 10]  KiVec=[5 5]  KgVec=[0 0]  vnom=5  Kaw=1  tauerr=.075  a=VEH.FrontAxlePositionfromCG  b=VEH.RearAxlePositionfromCG  m=VEH.Mass  I=VEH.YawMomentInertia  Cy_f=5000  Cy_r=7000  theta=40*pi/180  tau=0.03  L=1.0  Kpt=20000  aR=200  bR=2.5  cR=.5  g=9.81  GearInit=0  tShift=.1  pdlVec=[0.1 0.4 0.5 0.9]  upShftTbl=[-1 12.9375 26.4375 39.9375 51.18749999999999 62.4375 72.84375 83.25;-1 16.3125 29.8125 43.3125 54.5624 65.8125 76.78125 87.75;-1 19.6875 33.1875 46.68749999999999 57.9375 69.1875 80.71875 92.25;-1 33 52.5 77.25 100.5 138.75 161.875 185]  dwnShftTbl=[-1 12.9375 26.4375 39.9375 51.18749999999999 62.4375 72.84375 83.25;-1 16.3125 29.8125 43.3125 54.5624 65.8125 76.78125 87.75;-1 19.6875 33.1875 46.68749999999999 57.9375 69.1875 80.71875 92.25;-1 33 52.5 77.25 100.5 138.75 161.875 185]  tClutch=.5  tRev=.5  tPark=120  aMode=2  UpGearVec="[0  1  2  3  4  5  6  7]"  DownGearVec="[1  2  3  4  5  6  7  8]"
      link override Shift: LabelModeActiveChoice=0
      settings: SourceProductName=Vehicle Dynamics Blockset  SourceProductBaseCode=VE
  Switch : Switch  Criteria=u2 > Threshold
  Terminator : Terminator
  Wheel Angle Limit * Steer Ratio : Gain  Gain=20*pi/180*18
  Driver : Outport  VectorParamsAs1DForOutWhenUnconnected=off
  wires:
  Switch/1 -> Bus Creator1/2  "Accel"
  Linear Predictive Driver/2 -> Dead Zone1/1  "SteerCmd"
  Linear Predictive Driver/3 -> Switch/3  "AccelCmd"
  Bus Selector/3 -> Linear Predictive Driver/6  "<ydot>"
  Ground/1 -> Linear Predictive Driver/3
  Constant/1 -> Switch/1
  Bus Selector/1 -> Dead Zone/1  "<xdot>"
  Bus Selector/2 -> Linear Predictive Driver/5  "<Y>"
  Bus Selector1/3 -> Switch/2  "<ThrotKill>"
  Bus Creator1/1 -> Driver/1
  Dead Zone/1 -> Linear Predictive Driver/4
  Linear Predictive Driver/1 -> Terminator/1
  Bus Selector/4 -> Linear Predictive Driver/7  "<psi>"
  VehFdbk/1 -> Bus Selector/1
  Bus Selector1/2 -> Linear Predictive Driver/2  "<LtrlRef>"
  Bus Selector/5 -> Linear Predictive Driver/8  "<r>"
  Dead Zone1/1 -> Wheel Angle Limit * Steer Ratio/1
  VehRef/1 -> Bus Selector1/1
  Bus Selector1/1 -> Linear Predictive Driver/1  "<LngRef>"
  Wheel Angle Limit * Steer Ratio/1 -> Bus Creator1/1  "Steer"
  Linear Predictive Driver/4 -> Bus Creator1/3  "Brake"
  Linear Predictive Driver/5 -> Bus Creator1/4  "Gear"

== system car_model_PIL/Environment/Ground Feedback/3D Engine ==
  Friction : Inport
  Bus Creator : BusCreator  Inputs=4
  Bus Creator2 : BusCreator  Inputs=4
  Bus Creator3 : BusCreator  Inputs=2
  Bus Selector : BusSelector  OutputSignals=HitLoc
  Data Type Conversion : DataTypeConversion
  Demux : Demux
  Demux1 : Demux
  Passenger Vehicle Ray Trace Set : sim3dlib/Vehicle Terrain Sensor  ActorTag=SimulinkVehicle1  VehExtEn=Constant  TireRadiiExt=Constant  VehCntrLngthVal=0  TireRadiiVal=0  VehRayLngth=10  LfRayLngth=20  RfRayLngth=20  LrRayLngth=20  RrRayLngth=20  VehRayOffset=0  LfRayOffset=-1  RfRayOffset=-1  LrRayOffset=-1  RrRayOffset=-1  VehEn=on  LfEn=on  RfEn=on  LrEn=on  RrEn=on  DbgEn=off  Ts=.03  aMode=aMode
      settings: SourceProductName=Vehicle Dynamics Blockset  SourceProductBaseCode=VE
  Rate Transition : RateTransition
  Reshape10 : Reshape  OutputDimensionality=Row vector (2-D)
  Selector1 : Selector  InputPortWidth=5  IndexOptions=Index vector (dialog)  Indices=[2:5]  OutputSizes=1
  Signal Specification : SignalSpecification  Unit=m
  Signal Specification1 : SignalSpecification  Unit=1
  Terminator1 : Terminator
  Terminator2 : Terminator
  Zend Select : Selector  NumberOfDimensions=2  InputPortWidth=3  IndexOptions=Select all,Index vector (dialog)  Indices=[1 3],3  OutputSizes=1,1
  Ground : Outport  VectorParamsAs1DForOutWhenUnconnected=off
  wires:
  Selector1/1 -> Rate Transition/1
  Zend Select/1 -> Reshape10/1
  Bus Selector/1 -> Zend Select/1  "<HitLoc>"
  Passenger Vehicle Ray Trace Set/2 -> Terminator1/1
  Passenger Vehicle Ray Trace Set/3 -> Terminator2/1
  Reshape10/1 -> Selector1/1
  Passenger Vehicle Ray Trace Set/1 -> Bus Selector/1
  Rate Transition/1 -> Data Type Conversion/1
  Demux/2 -> Bus Creator/2  "G_FR_z"
  Demux/1 -> Bus Creator/1  "G_FL_z"
  Demux/4 -> Bus Creator/4  "G_RR_z"
  Demux/3 -> Bus Creator/3  "G_RL_z"
  Signal Specification/1 -> Demux/1
  Signal Specification1/1 -> Demux1/1
  Demux1/1 -> Bus Creator2/1  "mu_FL"
  Bus Creator/1 -> Bus Creator3/1  "z"
  Demux1/3 -> Bus Creator2/3  "mu_RL"
  Demux1/4 -> Bus Creator2/4  "mu_RR"
  Demux1/2 -> Bus Creator2/2  "mu_FR"
  Bus Creator2/1 -> Bus Creator3/2  "mu"
  Bus Creator3/1 -> Ground/1
  Friction/1 -> Signal Specification1/1
  Data Type Conversion/1 -> Signal Specification/1

== system car_model_PIL/Environment/Ground Feedback/Constant ==
  Friction : Inport
  Bus Creator : BusCreator  Inputs=4
  Bus Creator2 : BusCreator  Inputs=4
  Bus Creator3 : BusCreator  Inputs=2
  Constant1 : Constant  Value=zeros(4,1)
  Demux : Demux
  Demux1 : Demux
  Signal Specification : SignalSpecification  Unit=m
  Signal Specification1 : SignalSpecification  Unit=1
  Ground : Outport  VectorParamsAs1DForOutWhenUnconnected=off
  wires:
  Constant1/1 -> Signal Specification/1
  Signal Specification/1 -> Demux/1
  Demux/4 -> Bus Creator/4  "G_RR_z"
  Demux/1 -> Bus Creator/1  "G_FL_z"
  Demux/3 -> Bus Creator/3  "G_RL_z"
  Demux/2 -> Bus Creator/2  "G_FR_z"
  Bus Creator/1 -> Bus Creator3/1  "z"
  Demux1/3 -> Bus Creator2/3  "mu_RL"
  Demux1/4 -> Bus Creator2/4  "mu_RR"
  Demux1/1 -> Bus Creator2/1  "mu_FL"
  Demux1/2 -> Bus Creator2/2  "mu_FR"
  Bus Creator2/1 -> Bus Creator3/2  "mu"
  Friction/1 -> Signal Specification1/1
  Signal Specification1/1 -> Demux1/1
  Bus Creator3/1 -> Ground/1

== system car_model_PIL/Passenger Vehicle/Subsystem5/Brake Hydraulics1 ==
  BrkPrsCmd : Inport
  Circuit : Switch  Criteria=u2 ~= 0
  Constant : Constant  Value=-1
  Gain4 : Gain  Gain=8e6
  Valve : autolibutils/Cont LPF  wc=200*2*pi  aMode=2
      settings: SourceProductName=Powertrain Blockset  SourceProductBaseCode=PW
  Volume : Integrator  LimitOutput=on  UpperSaturationLimit=1  LowerSaturationLimit=0  AbsoluteTolerance=1e-3
  BrkPrs : Outport  VectorParamsAs1DForOutWhenUnconnected=off
  wires:
  Volume/1 -> Gain4/1
  Valve/1 -> Volume/1  "Flow"
  BrkPrsCmd/1 -> Circuit/1, Circuit/2
  Gain4/1 -> BrkPrs/1  "Pressure"
  Circuit/1 -> Valve/1
  Constant/1 -> Circuit/3

== system car_model_PIL/Passenger Vehicle/Subsystem6/Suspension ==
  Steering : Inport
  Vehicle : Inport  Port=2
  Wheel : Inport  Port=3
  Double Wishbone Suspension : Subsystem  VariantControl=1
      mask Display: image('suspdw.png');
  Independent Mapped Front Suspension Mapped Solid Axle Rear Suspension : Subsystem  VariantControl=2
      mask Display: image([imread('suspindmap.png');imread('suspsamap.png')]);
  MacPherson Front Suspension Solid Axle Rear Suspension : Subsystem  VariantControl=3
      mask Display: image([imread('suspmacp.png');imread('suspsacoil.png')]);
  MacPherson Suspension : Subsystem  VariantControl=4
      mask Display: image('suspmacp.png');
  Mapped Suspension : Subsystem  VariantControl=5
      mask Display: image('suspindmap.png');
  Suspension : Outport  VectorParamsAs1DForOutWhenUnconnected=off

== system car_model_PIL/Passenger Vehicle/Subsystem6/Vehicle ==
  Suspension : Inport
  Wind : Inport  Port=2
  Variant Subsystem : Subsystem  VariantControlMode=Label  Variant=on  LabelModeActiveChoice=1
  VehFdbk : Outport  VectorParamsAs1DForOutWhenUnconnected=off
  wires:
  Variant Subsystem/1(VehFdbk) -> VehFdbk/1  "VehFdbk"
  Wind/1 -> Variant Subsystem/2(Wind)
  Suspension/1 -> Variant Subsystem/1(Suspension)

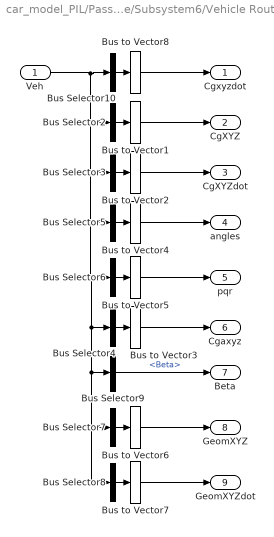
== system car_model_PIL/Passenger Vehicle/Subsystem6/Vehicle Routing ==
  Veh : Inport
  Bus Selector10 : BusSelector  OutputSignals=BdyFrm.Cg.Vel.xdot,BdyFrm.Cg.Vel.ydot,BdyFrm.Cg.Vel.zdot  OutputAsBus=on
  Bus Selector2 : BusSelector  OutputSignals=InertFrm.Cg.Disp.X,InertFrm.Cg.Disp.Y,InertFrm.Cg.Disp.Z  OutputAsBus=on
  Bus Selector3 : BusSelector  OutputSignals=InertFrm.Cg.Vel.Xdot,InertFrm.Cg.Vel.Ydot,InertFrm.Cg.Vel.Zdot  OutputAsBus=on
  Bus Selector4 : BusSelector  OutputSignals=BdyFrm.Cg.Acc.ax,BdyFrm.Cg.Acc.ay,BdyFrm.Cg.Acc.az  OutputAsBus=on
  Bus Selector5 : BusSelector  OutputSignals=InertFrm.Cg.Ang.phi,InertFrm.Cg.Ang.theta,InertFrm.Cg.Ang.psi  OutputAsBus=on
  Bus Selector6 : BusSelector  OutputSignals=BdyFrm.Cg.AngVel.p,BdyFrm.Cg.AngVel.q,BdyFrm.Cg.AngVel.r  OutputAsBus=on
  Bus Selector7 : BusSelector  OutputSignals=InertFrm.Geom.Disp.X,InertFrm.Geom.Disp.Y,InertFrm.Geom.Disp.Z  OutputAsBus=on
  Bus Selector8 : BusSelector  OutputSignals=InertFrm.Geom.Vel.Xdot,InertFrm.Geom.Vel.Ydot,InertFrm.Geom.Vel.Zdot  OutputAsBus=on
  Bus Selector9 : BusSelector  OutputSignals=BdyFrm.Geom.Ang.Beta
  Bus to Vector{1..8} (8 alike) : BusToVector
  Cgxyzdot : Outport  VectorParamsAs1DForOutWhenUnconnected=off
  CgXYZ : Outport  Port=2  VectorParamsAs1DForOutWhenUnconnected=off
  CgXYZdot : Outport  Port=3  VectorParamsAs1DForOutWhenUnconnected=off
  angles : Outport  Port=4  VectorParamsAs1DForOutWhenUnconnected=off
  pqr : Outport  Port=5  VectorParamsAs1DForOutWhenUnconnected=off
  Cgaxyz : Outport  Port=6  VectorParamsAs1DForOutWhenUnconnected=off
  Beta : Outport  Port=7  VectorParamsAs1DForOutWhenUnconnected=off
  GeomXYZ : Outport  Port=8  VectorParamsAs1DForOutWhenUnconnected=off
  GeomXYZdot : Outport  Port=9  VectorParamsAs1DForOutWhenUnconnected=off
  wires:
  Bus Selector3/1 -> Bus to Vector2/1
  Bus to Vector1/1 -> CgXYZ/1
  Bus to Vector5/1 -> pqr/1
  Bus Selector5/1 -> Bus to Vector4/1
  Bus Selector6/1 -> Bus to Vector5/1
  Bus to Vector4/1 -> angles/1
  Bus to Vector8/1 -> Cgxyzdot/1
  Bus Selector2/1 -> Bus to Vector1/1
  Bus Selector8/1 -> Bus to Vector7/1
  Bus to Vector6/1 -> GeomXYZ/1
  Bus Selector9/1 -> Beta/1  "<Beta>"
  Bus Selector4/1 -> Bus to Vector3/1
  Bus Selector10/1 -> Bus to Vector8/1
  Bus to Vector7/1 -> GeomXYZdot/1
  Bus to Vector3/1 -> Cgaxyz/1
  Bus Selector7/1 -> Bus to Vector6/1
  Bus to Vector2/1 -> CgXYZdot/1
  Veh/1 -> Bus Selector8/1, Bus Selector7/1, Bus Selector9/1, Bus Selector4/1, Bus Selector6/1, Bus Selector5/1, Bus Selector3/1, Bus Selector2/1, Bus Selector10/1
